simulink subsystem "HI_CAN"  (R2019b)
settings: Solver=VariableStepAuto  StartTime=0.0  StopTime=10.0  RelTol=1e-3
libraries: canmsglib x1, c280xlib x1
settings Model: Creator=Nick  LastModifiedBy=Nick

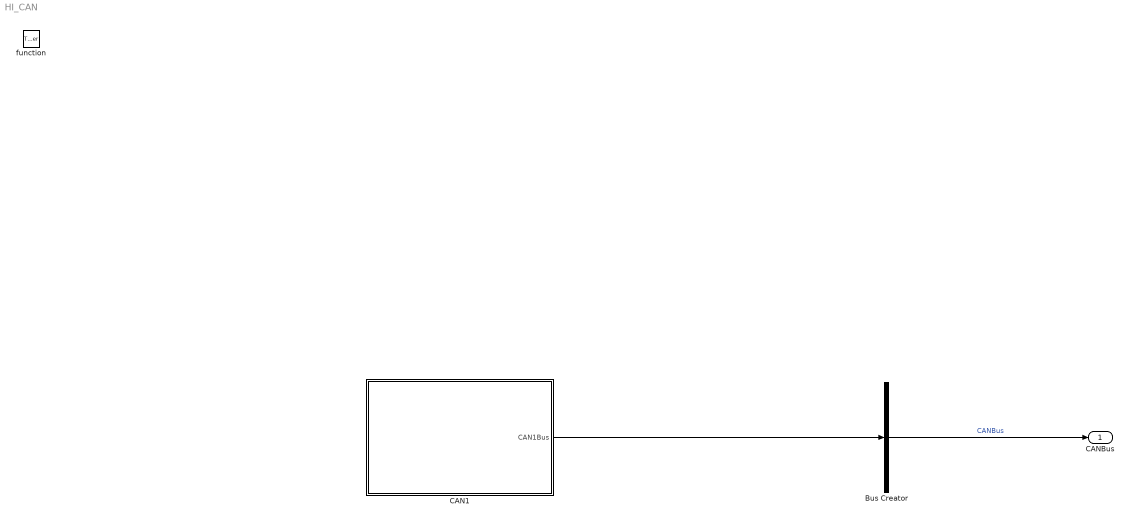
== system HI_CAN ==
  function : TriggerPort  TriggerType=function-call  VariantControl=Variant
  Bus Creator : BusCreator  Inputs=1
  CAN1 : Subsystem  TreatAsAtomicUnit=on
  CANBus : Outport
  wires:
  Bus Creator/1 -> CANBus/1  "CANBus"
  CAN1/1(CAN1Bus) -> Bus Creator/1

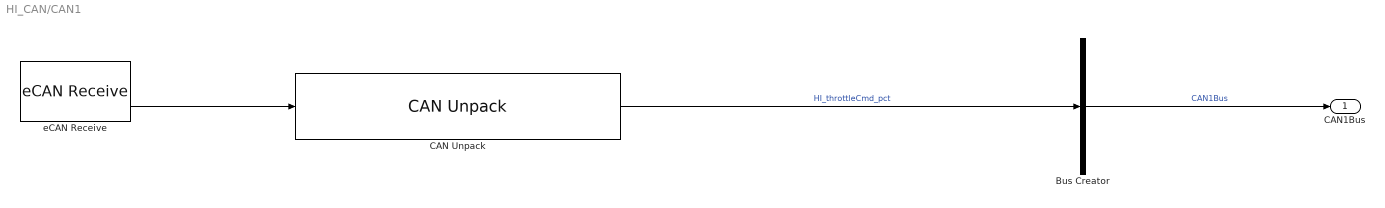
== system HI_CAN/CAN1 ==
  Bus Creator : BusCreator  Inputs=1
  CAN Unpack : canmsglib/CAN Unpack  CANdbFile=C:\Git\ETC-Development\DBCs\F28379D_etc_benchTest_CAN1.dbc  MsgList=USER_cmd1  MsgName=USER_cmd1  MsgIDType=Standard (11-bit identifier)  MsgIdentifier=500  MsgLength=2  SignalInfo={ 'USER_throttleCmd', '0', '16', 'LE', 'signed', 'Standard', '0', '0.01', '0', '-327.68', '327.67' }  IDPort=off  TimestampPort=off  ErrorPort=off  RemotePort=off  LengthPort=off  StatusPort=off  ApplyMinMax=off
      settings: SourceProductName=Vehicle Network Toolbox  SourceProductBaseCode=VN  DataFormat=CANdb specified signals
  eCAN Receive : c280xlib/eCAN Receive  chipFamily=C280x  useModule=eCAN_A  mailboxNo=3  messageID=500  messageType=Standard (11-bit identifier)  sampleTime=-1  dataType=CAN_MESSAGE_TYPE  initValue=0  outputMessageLength=off  outputMessageTimeStamp=off  postInterrupt=off  interruptLine=0
      settings: SourceProductName=Embedded Coder Support Package for Texas Instruments C2000 Processors  SourceProductBaseCode=TIC2000
  CAN1Bus : Outport
  wires:
  CAN Unpack/1 -> Bus Creator/1  "HI_throttleCmd_pct"
  eCAN Receive/2 -> CAN Unpack/1
  Bus Creator/1 -> CAN1Bus/1  "CAN1Bus"
